simulink model "Session3_PID_OS_simulink2"  (R2014a)
settings: Solver=ode45  StartTime=0.0  StopTime=60  RelTol=1e-3
libraries: simulink x2
settings Model: Creator=Omar Emad  LastModifiedBy=Omar Emad

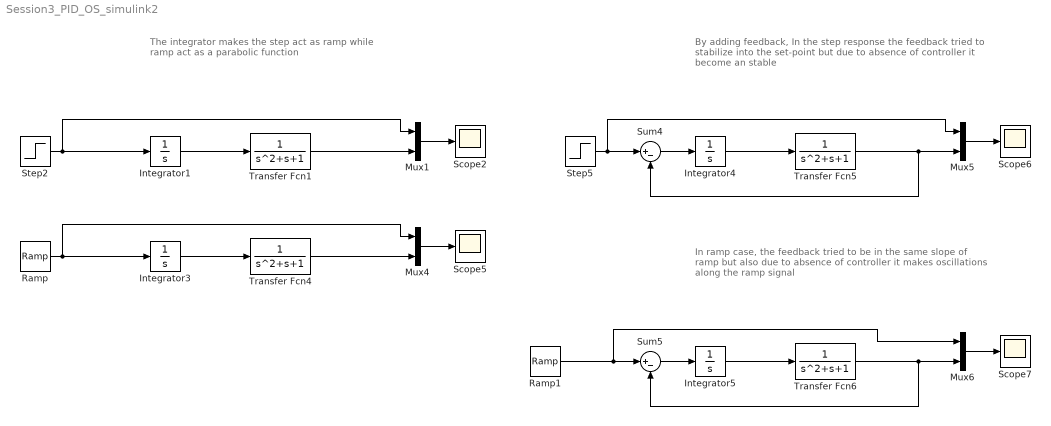
== system Session3_PID_OS_simulink2 ==
  note: The integrator makes  the step act as ramp
      | while ramp act as a parabolic function
  note: By adding feedback, In the step response the feedback
      | tried to stabilize into the set-point but due to absence of
      | controller it become an stable
  note: In ramp case, the feedback tried to be in the same slope
      | of ramp but also due to absence of controller it makes
      | oscillations along the ramp signal
  Integrator{1,3..5} (4 alike) : Integrator
  Mux{1,4..6} (4 alike) : Mux  Inputs=2
  Ramp : simulink/Sources/Ramp  slope=1  start=0  X0=0
  Ramp1 : simulink/Sources/Ramp  slope=1  start=0  X0=0
  Scope{2,5..7} (4 alike) : Scope
      Scope2 settings: SaveName=ScopeData2
      Scope5 settings: SaveName=ScopeData5
      Scope6 settings: SaveName=ScopeData6
      Scope7 settings: SaveName=ScopeData7
  Step2 : Step  SampleTime=0
  Step5 : Step  SampleTime=0
  Sum4 : Sum  Inputs=|+-
  Sum5 : Sum  Inputs=|+-
  Transfer Fcn{1,4..6} (4 alike) : TransferFcn  Denominator=[1 1 1]
  wires:
  Step2/1 -> Integrator1/1, Mux1/1
  Transfer Fcn1/1 -> Mux1/2
  Mux1/1 -> Scope2/1
  Integrator1/1 -> Transfer Fcn1/1
  Ramp/1 -> Mux4/1, Integrator3/1
  Transfer Fcn4/1 -> Mux4/2
  Mux4/1 -> Scope5/1
  Integrator3/1 -> Transfer Fcn4/1
  Step5/1 -> Sum4/1, Mux5/1
  Transfer Fcn5/1 -> Sum4/2, Mux5/2
  Mux5/1 -> Scope6/1
  Integrator4/1 -> Transfer Fcn5/1
  Sum4/1 -> Integrator4/1
  Ramp1/1 -> Sum5/1, Mux6/1
  Transfer Fcn6/1 -> Mux6/2, Sum5/2
  Mux6/1 -> Scope7/1
  Integrator5/1 -> Transfer Fcn6/1
  Sum5/1 -> Integrator5/1
